simulink model "pulse_heating_official_spine_v04_git_recovery"  (R2025b)
settings: Solver=VariableStepAuto  StartTime=0.0  StopTime=0.001  RelTol=1e-3
PreLoadFcn:
  | addpath('C:\Users\ADMIN\Documents\MATLAB\Examples\R2025b\simscapeelectrical\BatteryThermalManagementExample');
  | addpath('C:\Users\ADMIN\Documents\MATLAB\Examples\R2025b\mcb\SIUnitsExample');
  | addpath('C:\Users\ADMIN\Documents\MATLAB\Examples\R2025b\simscapeelectrical\PMSMDriveThermalExample');
  | load_system('PMSMDriveThermal');
  | set_param('PMSMDriveThermal','SimscapeLogType','none','SimscapeLogSimulationStatistics','off');
  | set_param('PMSMDriveThermal','Dirty','off');
InitFcn:
  | addpath('C:\Users\ADMIN\Documents\MATLAB\Examples\R2025b\simscapeelectrical\BatteryThermalManagementExample');
  | addpath('C:\Users\ADMIN\Documents\MATLAB\Examples\R2025b\mcb\SIUnitsExample');
  | addpath('C:\Users\ADMIN\Documents\MATLAB\Examples\R2025b\simscapeelectrical\PMSMDriveThermalExample');
  | load_system('PMSMDriveThermal');
  | PMSMDriveThermalData;
  | mcb_pmsm_foc_qep_f28379d_SIUnit_data;
  | bw_i = (PI_params.Kp_i + pmsm.Rs) / pmsm.Ld;
  | pmsm.Rs = Rs; pmsm.Ld = Ld; pmsm.Lq = Lq; pmsm.p = N; pmsm.FluxPM = PM;
  | pmsm.J = J; pmsm.Ke = PM*N; pmsm.Kt = 1.5*N*PM;
  | PI_params.Kp_i = bw_i * Ld - Rs; PI_params.Ki_i = bw_i * Rs; PI_params.Ti_i = 1/bw_i;
  | PI_params.Kp_id = PI_params.Kp_i; PI_params.Ki_id = PI_params.Ki_i; PI_params.Ti_id = PI_params.Ti_i;
  | inverter.V_dc = 70; dataType = 'double';
  | BatteryThermalManagementInitialization;
  | ambient=263.15; coolantTemp=263.15; cellT_ini=ambient*ones(1,Ns*Np); cellT_ini4=ambient*ones(1,Ns4*Np4);
model workspace (MAT data in the model file):
  control_status_v4d2_partial_duty_code = 6
  diagnostic_frequency_Hz = 50
  drive_status_v4d2_partial_current_code = 6
  kpi_status_v4d2_partial_numeric_code = 6
  kpi_value_unknown = nan
  limit_factor_unknown_code = 99
  limit_margin_unknown_value = nan
  limit_status_v4c_code = 5
  pulse_command_status_code = 6
  pulse_duty_percent = 50
  pulse_id_amplitude_A = 1
  pulse_iq_amplitude_A = 0
  pulse_mode_code = 4
  pulse_phase_delay_s = 0
undefined symbols (not defined in the file): DiscIntNeverNeededParam, f_losses, Flowrate_vec, fsw, Isc_losses, losses_oc, losses_sc, N, PM, Rs, Ts, Tsc
libraries: fl_lib x36, nesl_utility x33, ee_lib x9, mcbcontrolslib x5, mcbeeMathTransformLib x3, slpidlib x2, simulink x1
(part 2 of 4)

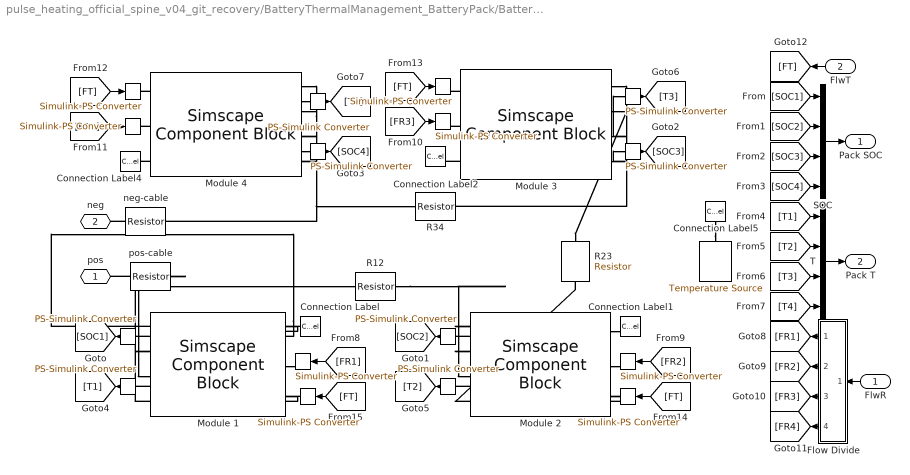
== system pulse_heating_official_spine_v04_git_recovery/BatteryThermalManagement_BatteryPack/Battery_pack ==
  FlwR : Inport
  FlwT : Inport  Port=2
  " " : nesl_utility/PS-Simulink Converter  PhysicalDomain=network_engine_domain  SubClassName=ps_output  LeftPortType=input  RightPortType=output  PseudoPeriodic=off  Frequencies=[]  VectorFormat=1-D array  Unit=inherit  AffineConversion=off
  "  " : nesl_utility/PS-Simulink Converter  PhysicalDomain=network_engine_domain  SubClassName=ps_output  LeftPortType=input  RightPortType=output  PseudoPeriodic=off  Frequencies=[]  VectorFormat=1-D array  Unit=inherit  AffineConversion=off
  "   " : nesl_utility/PS-Simulink Converter  PhysicalDomain=network_engine_domain  SubClassName=ps_output  LeftPortType=input  RightPortType=output  PseudoPeriodic=off  Frequencies=[]  VectorFormat=1-D array  Unit=inherit  AffineConversion=off
  "    " : nesl_utility/Simulink-PS Converter  PhysicalDomain=network_engine_domain  SubClassName=ps_input  LeftPortType=input  RightPortType=output  PseudoPeriodic=off  Frequencies=[]  NoiseDistribution=none  NoiseParameters=[]  Unit=1  AffineConversion=off  FilteringAndDerivatives=filter  SimscapeFilterOrder=1  InputFilterTimeConstant=0.01  UdotUserProvided=0
  "     " : fl_lib/Thermal/Thermal Sources/Temperature Source  temperature=ambient K
  "      " : nesl_utility/PS-Simulink Converter  PhysicalDomain=network_engine_domain  SubClassName=ps_output  LeftPortType=input  RightPortType=output  PseudoPeriodic=off  Frequencies=[]  VectorFormat=1-D array  Unit=inherit  AffineConversion=off
  "       " : nesl_utility/Simulink-PS Converter  PhysicalDomain=network_engine_domain  SubClassName=ps_input  LeftPortType=input  RightPortType=output  PseudoPeriodic=off  Frequencies=[]  NoiseDistribution=none  NoiseParameters=[]  Unit=1  AffineConversion=off  FilteringAndDerivatives=filter  SimscapeFilterOrder=1  InputFilterTimeConstant=0.01  UdotUserProvided=0
  "         " : nesl_utility/PS-Simulink Converter  PhysicalDomain=network_engine_domain  SubClassName=ps_output  LeftPortType=input  RightPortType=output  PseudoPeriodic=off  Frequencies=[]  VectorFormat=1-D array  Unit=inherit  AffineConversion=off
  "          " : nesl_utility/PS-Simulink Converter  PhysicalDomain=network_engine_domain  SubClassName=ps_output  LeftPortType=input  RightPortType=output  PseudoPeriodic=off  Frequencies=[]  VectorFormat=1-D array  Unit=inherit  AffineConversion=off
  "           " : nesl_utility/Simulink-PS Converter  PhysicalDomain=network_engine_domain  SubClassName=ps_input  LeftPortType=input  RightPortType=output  PseudoPeriodic=off  Frequencies=[]  NoiseDistribution=none  NoiseParameters=[]  Unit=1  AffineConversion=off  FilteringAndDerivatives=filter  SimscapeFilterOrder=1  InputFilterTimeConstant=0.01  UdotUserProvided=0
  "            " : nesl_utility/PS-Simulink Converter  PhysicalDomain=network_engine_domain  SubClassName=ps_output  LeftPortType=input  RightPortType=output  PseudoPeriodic=off  Frequencies=[]  VectorFormat=1-D array  Unit=inherit  AffineConversion=off
  "              " : nesl_utility/Simulink-PS Converter  PhysicalDomain=network_engine_domain  SubClassName=ps_input  LeftPortType=input  RightPortType=output  PseudoPeriodic=off  Frequencies=[]  NoiseDistribution=none  NoiseParameters=[]  Unit=1  AffineConversion=off  FilteringAndDerivatives=filter  SimscapeFilterOrder=1  InputFilterTimeConstant=0.01  UdotUserProvided=0
  "               " : nesl_utility/Simulink-PS Converter  PhysicalDomain=network_engine_domain  SubClassName=ps_input  LeftPortType=input  RightPortType=output  PseudoPeriodic=off  Frequencies=[]  NoiseDistribution=none  NoiseParameters=[]  Unit=1  AffineConversion=off  FilteringAndDerivatives=filter  SimscapeFilterOrder=1  InputFilterTimeConstant=0.01  UdotUserProvided=0
  "                      " : nesl_utility/Simulink-PS Converter  PhysicalDomain=network_engine_domain  SubClassName=ps_input  LeftPortType=input  RightPortType=output  PseudoPeriodic=off  Frequencies=[]  NoiseDistribution=none  NoiseParameters=[]  Unit=1  AffineConversion=off  FilteringAndDerivatives=filter  SimscapeFilterOrder=1  InputFilterTimeConstant=0.01  UdotUserProvided=0
  "                                      " : nesl_utility/PS-Simulink Converter  PhysicalDomain=network_engine_domain  SubClassName=ps_output  LeftPortType=input  RightPortType=output  PseudoPeriodic=off  Frequencies=[]  VectorFormat=1-D array  Unit=inherit  AffineConversion=off
  "                                           " : nesl_utility/Simulink-PS Converter  PhysicalDomain=network_engine_domain  SubClassName=ps_input  LeftPortType=input  RightPortType=output  PseudoPeriodic=off  Frequencies=[]  NoiseDistribution=none  NoiseParameters=[]  Unit=1  AffineConversion=off  FilteringAndDerivatives=filter  SimscapeFilterOrder=1  InputFilterTimeConstant=0.01  UdotUserProvided=0
  "                                                  " : nesl_utility/Simulink-PS Converter  PhysicalDomain=network_engine_domain  SubClassName=ps_input  LeftPortType=input  RightPortType=output  PseudoPeriodic=off  Frequencies=[]  NoiseDistribution=none  NoiseParameters=[]  Unit=1  AffineConversion=off  FilteringAndDerivatives=filter  SimscapeFilterOrder=1  InputFilterTimeConstant=0.01  UdotUserProvided=0
  "                        Flow Divide" : Subsystem
  Connection Label{,1..2,4..5} (5 alike) : ConnectionLabel  Label=Amb
  Module 1 : SimscapeComponentBlock  SourceFile=BatteryModule  ComponentPath=BatteryModule  ComponentVariants="[\"BatteryModule\"]"  ComponentVariantNames="[\"BatteryModule\"]"  ClassName=BatteryModule  SchemaVersion=1  LUTpointsTemp=T_vec K  cellAH=AH A*hr  LUTpointsSOC=SOC_vec  LUTpointsFlowrate=Flowrate_vec kg/s  V0_mat=V0_mat V  prm_dir=simscape.enum.tablebattery.prm_dir.noCurrentDirectionality  R0_mat=R0_mat Ohm  R0_dis_mat=[.03, .015, .002; .04, .017, .008; .039, .012, .006; .027, .013, .021] Ohm  R0_ch_mat=[.03, .015, .002; .04, .017, .008; .039, .012, .006; .027, .013, .021] Ohm  prm_leak=simscape.enum.tablebattery.prm_leak.disabled  Rleak_vec=Rleak Ohm  extrapolation_option=simscape.enum.extrapolation.nearest  prm_dyn=simscape.enum.tablebattery.prm_dyn.rc2  R1_mat=R1_mat Ohm  tau1_mat=Tau1_mat s  R2_mat=R2_mat Ohm  tau2_mat=Tau2_mat s  R3_mat=[.014, .382, .407; .028, .006, .007; .014, .007, .006; .333, .956, .912] Ohm  tau3_mat=[1, 44, 5644; 11, 24, 506; 2, 14, 330; 3310, 13419, 30216] s  R4_mat=[.014, .382, .407; .028, .006, .007; .014, .007, .006; .333, .956, .912] Ohm  tau4_mat=[1, 44, 5644; 11, 24, 506; 2, 14, 330; 3310, 13419, 30216] s  R5_mat=[.014, .382, .407; .028, .006, .007; .014, .007, .006; .333, .956, .912] Ohm  tau5_mat=[1, 44, 5644; 11, 24, 506; 2, 14, 330; 3310, 13419, 30216] s  prm_fade=simscape.enum.tablebattery.prm_fade.equations  N0=Ndisc  dV0=delV0  dR0=delR0  dAH=delAH  dRleak=delLeak  dR1=delR1  dR2=delR2  dR3=0  dR4=0  dR5=0  N0vec=[100, 200, 300]  Tfadevec=[298.15, 323.15] K  dV0vec=[0, 0, 0]  dR0vec=[0, 0, 0]  dAHvec=[0, 0, 0]  dRleakvec=[0, 0, 0]  dR1vec=[0, 0, 0]  dR2vec=[0, 0, 0]  dR3vec=[0, 0, 0]  dR4vec=[0, 0, 0]  dR5vec=[0, 0, 0]  dV0mat=[0, 0; 0, 0; 0, 0]  dR0mat=[0, 0; 0, 0; 0, 0]  dAHmat=[0, 0; 0, 0; 0, 0]  dRleakmat=[0, 0; 0, 0; 0, 0]  dR1mat=[0, 0; 0, 0; 0, 0]  dR2mat=[0, 0; 0, 0; 0, 0]  dR3mat=[0, 0; 0, 0; 0, 0]  dR4mat=[0, 0; 0, 0; 0, 0]  dR5mat=[0, 0; 0, 0; 0, 0]  cellThermalMass=MdotCp J/K  cellThermalCond=K_cell W/(m*K)  cellHeatTrCoeff=h_cell W/(m^2*K)  Ns=Ns  Np=Np  cellTypeSelection=BatteryTypeSelection.Pouch  cellHeight=cell_H m  cellWidth=cell_W m  cellThickness=cell_T m  cellDiameter=0.018 m  cellCylinLine=3  moduleExternalR=Rext Ohm  moduleCellBalancing=BatteryCellBalancingEnum.None  passiveShuntR=shuntR Ohm  passiveSWclosedR=swClosedR Ohm  passiveSWopenCond=swOpenC 1/Ohm  passiveSWthreshold=swThreshold  moduleCooling=coolantQ W/K  moduleExtHeat=extHeat W  cellTemp=cellT_ini K  cellSOC=cellSOC_ini  moduleCellAHpercentVar=AhrVar  moduleCellLeakPercentVar=RleakVar
      settings: CopyFcn=simscape.sscblock.internal.componentBlockCallback(gcbh,'COPY')  PreCopyFcn=simscape.sscblock.internal.componentBlockCallback(gcbh,'PRECOPY')  PreDeleteFcn=simscape.sscblock.internal.componentBlockCallback(gcbh,'PREDELETE')  InternalSimscapePortConfiguration="{\"Bottom\":[],\"Left\":[{\"id\":\"outputCellSOC\",\"label\":\"SOC\",\"type\":\"output\"},{\"id\":\"outputCellTemp\",\"label\":\"Temp\",\"type\":\"output\"}],\"Right\":[{\"id\":\"H\",\"label\":\"Amb\",\"type\":\"foundation.thermal.thermal\"},{\"id\":\"frac\",\"label\":\"FlwR\",\"type\":\"input\"},{\"id\":\"delT\",\"label\":\"FlwT\",\"type\":\"input\"}],\"Top\":[{\"id\":\"p\",\"label\":\"pos\",\"type\":\"foundation.electrical.electrical\"},{\"id\":\"n\",\"label\":\"neg\",\"type\":\"foundation.electrical.electrical\"}]}"
      mask Type: Battery Module
  Module 2 : SimscapeComponentBlock  SourceFile=BatteryModule  ComponentPath=BatteryModule  ComponentVariants="[\"BatteryModule\"]"  ComponentVariantNames="[\"BatteryModule\"]"  ClassName=BatteryModule  SchemaVersion=1  LUTpointsTemp=T_vec K  cellAH=AH A*hr  LUTpointsSOC=SOC_vec  LUTpointsFlowrate=Flowrate_vec kg/s  V0_mat=V0_mat V  prm_dir=simscape.enum.tablebattery.prm_dir.noCurrentDirectionality  R0_mat=R0_mat Ohm  R0_dis_mat=[.03, .015, .002; .04, .017, .008; .039, .012, .006; .027, .013, .021] Ohm  R0_ch_mat=[.03, .015, .002; .04, .017, .008; .039, .012, .006; .027, .013, .021] Ohm  prm_leak=simscape.enum.tablebattery.prm_leak.disabled  Rleak_vec=Rleak Ohm  extrapolation_option=simscape.enum.extrapolation.nearest  prm_dyn=simscape.enum.tablebattery.prm_dyn.rc2  R1_mat=R1_mat Ohm  tau1_mat=Tau1_mat s  R2_mat=R2_mat Ohm  tau2_mat=Tau2_mat s  R3_mat=[.014, .382, .407; .028, .006, .007; .014, .007, .006; .333, .956, .912] Ohm  tau3_mat=[1, 44, 5644; 11, 24, 506; 2, 14, 330; 3310, 13419, 30216] s  R4_mat=[.014, .382, .407; .028, .006, .007; .014, .007, .006; .333, .956, .912] Ohm  tau4_mat=[1, 44, 5644; 11, 24, 506; 2, 14, 330; 3310, 13419, 30216] s  R5_mat=[.014, .382, .407; .028, .006, .007; .014, .007, .006; .333, .956, .912] Ohm  tau5_mat=[1, 44, 5644; 11, 24, 506; 2, 14, 330; 3310, 13419, 30216] s  prm_fade=simscape.enum.tablebattery.prm_fade.equations  N0=Ndisc  dV0=delV0  dR0=delR0  dAH=delAH  dRleak=delLeak  dR1=delR1  dR2=delR2  dR3=0  dR4=0  dR5=0  N0vec=[100, 200, 300]  Tfadevec=[298.15, 323.15] K  dV0vec=[0, 0, 0]  dR0vec=[0, 0, 0]  dAHvec=[0, 0, 0]  dRleakvec=[0, 0, 0]  dR1vec=[0, 0, 0]  dR2vec=[0, 0, 0]  dR3vec=[0, 0, 0]  dR4vec=[0, 0, 0]  dR5vec=[0, 0, 0]  dV0mat=[0, 0; 0, 0; 0, 0]  dR0mat=[0, 0; 0, 0; 0, 0]  dAHmat=[0, 0; 0, 0; 0, 0]  dRleakmat=[0, 0; 0, 0; 0, 0]  dR1mat=[0, 0; 0, 0; 0, 0]  dR2mat=[0, 0; 0, 0; 0, 0]  dR3mat=[0, 0; 0, 0; 0, 0]  dR4mat=[0, 0; 0, 0; 0, 0]  dR5mat=[0, 0; 0, 0; 0, 0]  cellThermalMass=MdotCp J/K  cellThermalCond=K_cell W/(m*K)  cellHeatTrCoeff=h_cell W/(m^2*K)  Ns=Ns  Np=Np  cellTypeSelection=BatteryTypeSelection.Pouch  cellHeight=cell_H m  cellWidth=cell_W m  cellThickness=cell_T m  cellDiameter=0.018 m  cellCylinLine=3  moduleExternalR=Rext Ohm  moduleCellBalancing=BatteryCellBalancingEnum.None  passiveShuntR=shuntR Ohm  passiveSWclosedR=swClosedR Ohm  passiveSWopenCond=swOpenC 1/Ohm  passiveSWthreshold=swThreshold  moduleCooling=coolantQ W/K  moduleExtHeat=extHeat W  cellTemp=cellT_ini K  cellSOC=cellSOC_ini  moduleCellAHpercentVar=AhrVar  moduleCellLeakPercentVar=RleakVar
      settings: CopyFcn=simscape.sscblock.internal.componentBlockCallback(gcbh,'COPY')  PreCopyFcn=simscape.sscblock.internal.componentBlockCallback(gcbh,'PRECOPY')  PreDeleteFcn=simscape.sscblock.internal.componentBlockCallback(gcbh,'PREDELETE')  InternalSimscapePortConfiguration="{\"Bottom\":[],\"Left\":[{\"id\":\"outputCellSOC\",\"label\":\"SOC\",\"type\":\"output\"},{\"id\":\"outputCellTemp\",\"label\":\"Temp\",\"type\":\"output\"}],\"Right\":[{\"id\":\"H\",\"label\":\"Amb\",\"type\":\"foundation.thermal.thermal\"},{\"id\":\"frac\",\"label\":\"FlwR\",\"type\":\"input\"},{\"id\":\"delT\",\"label\":\"FlwT\",\"type\":\"input\"}],\"Top\":[{\"id\":\"p\",\"label\":\"pos\",\"type\":\"foundation.electrical.electrical\"},{\"id\":\"n\",\"label\":\"neg\",\"type\":\"foundation.electrical.electrical\"}]}"
      mask Type: Battery Module
  Module 3 : SimscapeComponentBlock  SourceFile=BatteryModule  ComponentPath=BatteryModule  ComponentVariants="[\"BatteryModule\"]"  ComponentVariantNames="[\"BatteryModule\"]"  ClassName=BatteryModule  SchemaVersion=1  LUTpointsTemp=T_vec K  cellAH=AH A*hr  LUTpointsSOC=SOC_vec  LUTpointsFlowrate=Flowrate_vec kg/s  V0_mat=V0_mat V  prm_dir=simscape.enum.tablebattery.prm_dir.noCurrentDirectionality  R0_mat=R0_mat Ohm  R0_dis_mat=[.03, .015, .002; .04, .017, .008; .039, .012, .006; .027, .013, .021] Ohm  R0_ch_mat=[.03, .015, .002; .04, .017, .008; .039, .012, .006; .027, .013, .021] Ohm  prm_leak=simscape.enum.tablebattery.prm_leak.disabled  Rleak_vec=Rleak Ohm  extrapolation_option=simscape.enum.extrapolation.nearest  prm_dyn=simscape.enum.tablebattery.prm_dyn.rc2  R1_mat=R1_mat Ohm  tau1_mat=Tau1_mat s  R2_mat=R2_mat Ohm  tau2_mat=Tau2_mat s  R3_mat=[.014, .382, .407; .028, .006, .007; .014, .007, .006; .333, .956, .912] Ohm  tau3_mat=[1, 44, 5644; 11, 24, 506; 2, 14, 330; 3310, 13419, 30216] s  R4_mat=[.014, .382, .407; .028, .006, .007; .014, .007, .006; .333, .956, .912] Ohm  tau4_mat=[1, 44, 5644; 11, 24, 506; 2, 14, 330; 3310, 13419, 30216] s  R5_mat=[.014, .382, .407; .028, .006, .007; .014, .007, .006; .333, .956, .912] Ohm  tau5_mat=[1, 44, 5644; 11, 24, 506; 2, 14, 330; 3310, 13419, 30216] s  prm_fade=simscape.enum.tablebattery.prm_fade.equations  N0=Ndisc  dV0=delV0  dR0=delR0  dAH=delAH  dRleak=delLeak  dR1=delR1  dR2=delR2  dR3=0  dR4=0  dR5=0  N0vec=[100, 200, 300]  Tfadevec=[298.15, 323.15] K  dV0vec=[0, 0, 0]  dR0vec=[0, 0, 0]  dAHvec=[0, 0, 0]  dRleakvec=[0, 0, 0]  dR1vec=[0, 0, 0]  dR2vec=[0, 0, 0]  dR3vec=[0, 0, 0]  dR4vec=[0, 0, 0]  dR5vec=[0, 0, 0]  dV0mat=[0, 0; 0, 0; 0, 0]  dR0mat=[0, 0; 0, 0; 0, 0]  dAHmat=[0, 0; 0, 0; 0, 0]  dRleakmat=[0, 0; 0, 0; 0, 0]  dR1mat=[0, 0; 0, 0; 0, 0]  dR2mat=[0, 0; 0, 0; 0, 0]  dR3mat=[0, 0; 0, 0; 0, 0]  dR4mat=[0, 0; 0, 0; 0, 0]  dR5mat=[0, 0; 0, 0; 0, 0]  cellThermalMass=MdotCp J/K  cellThermalCond=K_cell W/(m*K)  cellHeatTrCoeff=h_cell W/(m^2*K)  Ns=Ns  Np=Np  cellTypeSelection=BatteryTypeSelection.Pouch  cellHeight=cell_H m  cellWidth=cell_W m  cellThickness=cell_T m  cellDiameter=0.018 m  cellCylinLine=3  moduleExternalR=Rext Ohm  moduleCellBalancing=BatteryCellBalancingEnum.None  passiveShuntR=shuntR Ohm  passiveSWclosedR=swClosedR Ohm  passiveSWopenCond=swOpenC 1/Ohm  passiveSWthreshold=swThreshold  moduleCooling=coolantQ W/K  moduleExtHeat=extHeat W  cellTemp=cellT_ini K  cellSOC=cellSOC_ini  moduleCellAHpercentVar=AhrVar  moduleCellLeakPercentVar=RleakVar
      settings: CopyFcn=simscape.sscblock.internal.componentBlockCallback(gcbh,'COPY')  PreCopyFcn=simscape.sscblock.internal.componentBlockCallback(gcbh,'PRECOPY')  PreDeleteFcn=simscape.sscblock.internal.componentBlockCallback(gcbh,'PREDELETE')  InternalSimscapePortConfiguration="{\"Bottom\":[],\"Left\":[{\"id\":\"outputCellSOC\",\"label\":\"SOC\",\"type\":\"output\"},{\"id\":\"outputCellTemp\",\"label\":\"Temp\",\"type\":\"output\"}],\"Right\":[{\"id\":\"H\",\"label\":\"Amb\",\"type\":\"foundation.thermal.thermal\"},{\"id\":\"frac\",\"label\":\"FlwR\",\"type\":\"input\"},{\"id\":\"delT\",\"label\":\"FlwT\",\"type\":\"input\"}],\"Top\":[{\"id\":\"p\",\"label\":\"pos\",\"type\":\"foundation.electrical.electrical\"},{\"id\":\"n\",\"label\":\"neg\",\"type\":\"foundation.electrical.electrical\"}]}"
      mask Type: Battery Module
  Module 4 : SimscapeComponentBlock  SourceFile=BatteryModule  ComponentPath=BatteryModule  ComponentVariants="[\"BatteryModule\"]"  ComponentVariantNames="[\"BatteryModule\"]"  ClassName=BatteryModule  SchemaVersion=1  LUTpointsTemp=T_vec K  cellAH=AH A*hr  LUTpointsSOC=SOC_vec  LUTpointsFlowrate=Flowrate_vec kg/s  V0_mat=V0_mat V  prm_dir=simscape.enum.tablebattery.prm_dir.noCurrentDirectionality  R0_mat=R0_mat Ohm  R0_dis_mat=[.03, .015, .002; .04, .017, .008; .039, .012, .006; .027, .013, .021] Ohm  R0_ch_mat=[.03, .015, .002; .04, .017, .008; .039, .012, .006; .027, .013, .021] Ohm  prm_leak=simscape.enum.tablebattery.prm_leak.disabled  Rleak_vec=Rleak Ohm  extrapolation_option=simscape.enum.extrapolation.nearest  prm_dyn=simscape.enum.tablebattery.prm_dyn.rc2  R1_mat=R1_mat Ohm  tau1_mat=Tau1_mat s  R2_mat=R2_mat Ohm  tau2_mat=Tau2_mat s  R3_mat=[.014, .382, .407; .028, .006, .007; .014, .007, .006; .333, .956, .912] Ohm  tau3_mat=[1, 44, 5644; 11, 24, 506; 2, 14, 330; 3310, 13419, 30216] s  R4_mat=[.014, .382, .407; .028, .006, .007; .014, .007, .006; .333, .956, .912] Ohm  tau4_mat=[1, 44, 5644; 11, 24, 506; 2, 14, 330; 3310, 13419, 30216] s  R5_mat=[.014, .382, .407; .028, .006, .007; .014, .007, .006; .333, .956, .912] Ohm  tau5_mat=[1, 44, 5644; 11, 24, 506; 2, 14, 330; 3310, 13419, 30216] s  prm_fade=simscape.enum.tablebattery.prm_fade.equations  N0=Ndisc  dV0=delV0  dR0=delR0  dAH=delAH  dRleak=delLeak  dR1=delR1  dR2=delR2  dR3=0  dR4=0  dR5=0  N0vec=[100, 200, 300]  Tfadevec=[298.15, 323.15] K  dV0vec=[0, 0, 0]  dR0vec=[0, 0, 0]  dAHvec=[0, 0, 0]  dRleakvec=[0, 0, 0]  dR1vec=[0, 0, 0]  dR2vec=[0, 0, 0]  dR3vec=[0, 0, 0]  dR4vec=[0, 0, 0]  dR5vec=[0, 0, 0]  dV0mat=[0, 0; 0, 0; 0, 0]  dR0mat=[0, 0; 0, 0; 0, 0]  dAHmat=[0, 0; 0, 0; 0, 0]  dRleakmat=[0, 0; 0, 0; 0, 0]  dR1mat=[0, 0; 0, 0; 0, 0]  dR2mat=[0, 0; 0, 0; 0, 0]  dR3mat=[0, 0; 0, 0; 0, 0]  dR4mat=[0, 0; 0, 0; 0, 0]  dR5mat=[0, 0; 0, 0; 0, 0]  cellThermalMass=MdotCp J/K  cellThermalCond=K_cell W/(m*K)  cellHeatTrCoeff=h_cell W/(m^2*K)  Ns=Ns4  Np=Np4  cellTypeSelection=BatteryTypeSelection.Pouch  cellHeight=cell_H m  cellWidth=cell_W m  cellThickness=cell_T m  cellDiameter=0.018 m  cellCylinLine=3  moduleExternalR=Rext4 Ohm  moduleCellBalancing=BatteryCellBalancingEnum.None  passiveShuntR=shuntR Ohm  passiveSWclosedR=swClosedR Ohm  passiveSWopenCond=swOpenC 1/Ohm  passiveSWthreshold=swThreshold  moduleCooling=coolantQ4 W/K  moduleExtHeat=extHeat4 W  cellTemp=cellT_ini4 K  cellSOC=cellSOC_ini4  moduleCellAHpercentVar=AhrVar4  moduleCellLeakPercentVar=RleakVar
      settings: CopyFcn=simscape.sscblock.internal.componentBlockCallback(gcbh,'COPY')  PreCopyFcn=simscape.sscblock.internal.componentBlockCallback(gcbh,'PRECOPY')  PreDeleteFcn=simscape.sscblock.internal.componentBlockCallback(gcbh,'PREDELETE')  InternalSimscapePortConfiguration="{\"Bottom\":[],\"Left\":[{\"id\":\"outputCellSOC\",\"label\":\"SOC\",\"type\":\"output\"},{\"id\":\"outputCellTemp\",\"label\":\"Temp\",\"type\":\"output\"}],\"Right\":[{\"id\":\"H\",\"label\":\"Amb\",\"type\":\"foundation.thermal.thermal\"},{\"id\":\"frac\",\"label\":\"FlwR\",\"type\":\"input\"},{\"id\":\"delT\",\"label\":\"FlwT\",\"type\":\"input\"}],\"Top\":[{\"id\":\"p\",\"label\":\"pos\",\"type\":\"foundation.electrical.electrical\"},{\"id\":\"n\",\"label\":\"neg\",\"type\":\"foundation.electrical.electrical\"}]}"
      mask Type: Battery Module
  R12 : fl_lib/Electrical/Electrical Elements/Resistor  R=0.001 Ohm  i_specify=off  i_priority=None  i=0 A  i_nominal_specify=off  i_nominal_value=1  i_nominal_unit=A  v_specify=off  v_priority=None  v=0 V  v_nominal_specify=off  v_nominal_value=1  v_nominal_unit=V
  R23 : fl_lib/Electrical/Electrical Elements/Resistor  R=0.001 Ohm  i_specify=off  i_priority=None  i=0 A  i_nominal_specify=off  i_nominal_value=1  i_nominal_unit=A  v_specify=off  v_priority=None  v=0 V  v_nominal_specify=off  v_nominal_value=1  v_nominal_unit=V
  R34 : fl_lib/Electrical/Electrical Elements/Resistor  R=0.001 Ohm  i_specify=off  i_priority=None  i=0 A  i_nominal_specify=off  i_nominal_value=1  i_nominal_unit=A  v_specify=off  v_priority=None  v=0 V  v_nominal_specify=off  v_nominal_value=1  v_nominal_unit=V
  SOC : Concatenate  NumInputs=4
  T : Concatenate  NumInputs=4
  neg-cable : fl_lib/Electrical/Electrical Elements/Resistor  R=0.001 Ohm  i_specify=off  i_priority=None  i=0 A  i_nominal_specify=off  i_nominal_value=1  i_nominal_unit=A  v_specify=off  v_priority=None  v=0 V  v_nominal_specify=off  v_nominal_value=1  v_nominal_unit=V
  pos-cable : fl_lib/Electrical/Electrical Elements/Resistor  R=0.001 Ohm  i_specify=off  i_priority=None  i=0 A  i_nominal_specify=off  i_nominal_value=1  i_nominal_unit=A  v_specify=off  v_priority=None  v=0 V  v_nominal_specify=off  v_nominal_value=1  v_nominal_unit=V
  pos : PMIOPort  Side=Left
  neg : PMIOPort  Port=2  Side=Right
  Pack SOC : Outport
  Pack T : Outport  Port=2
  wires:
  "                        Flow Divide"/4(Out4) -> [FR4]
  "                        Flow Divide"/3(Out3) -> [FR3]
  "                        Flow Divide"/2(Out2) -> [FR2]
  "                        Flow Divide"/1(Out1) -> [FR1]
  FlwR/1 -> "                        Flow Divide"/1(In1)
  T/1 -> Pack T/1
  SOC/1 -> Pack SOC/1
  FlwT/1 -> [FT]
  [FT] -> "                                           "/1
  [FT] -> "                                                  "/1
  [FT] -> "              "/1
  [FT] -> "               "/1
  [FR4] -> "           "/1
  [FR3] -> "                      "/1
  [FR2] -> "       "/1
  [FR1] -> "    "/1
  "                                      "/1 -> [T4]
  "         "/1 -> [T3]
  "   "/1 -> [T2]
  " "/1 -> [T1]
  [T1] -> T/1
  [T2] -> T/2
  [T4] -> T/4
  [T3] -> T/3
  [SOC4] -> SOC/4
  [SOC3] -> SOC/3
  [SOC2] -> SOC/2
  [SOC1] -> SOC/1
  "            "/1 -> [SOC4]
  "          "/1 -> [SOC3]
  "      "/1 -> [SOC2]
  "  "/1 -> [SOC1]
  connections:
  pos-cable/RConn1 -- Module 1/LConn3
  pos-cable/LConn1 -- pos/RConn1
  Module 4/LConn4 -- neg-cable/LConn1
  neg-cable/RConn1 -- neg/RConn1
  Module 2/LConn4 -- R23/LConn1
  Module 3/LConn3 -- R23/RConn1
  Module 4/LConn3 -- R34/RConn1
  Module 3/LConn4 -- R34/LConn1
  R12/RConn1 -- Module 2/LConn3
  Module 1/LConn4 -- R12/LConn1
  "                                           "/RConn1 -- Module 1/RConn3
  "                                                  "/RConn1 -- Module 2/RConn3
  Module 1/RConn2 -- "    "/RConn1
  Connection Label5/LConn1 -- "     "/LConn1
  Module 4/RConn1 -- Connection Label4/LConn1
  Module 3/RConn1 -- Connection Label2/LConn1
  Module 2/RConn1 -- Connection Label1/LConn1
  Connection Label/LConn1 -- Module 1/RConn1
  Module 3/LConn2 -- "         "/LConn1
  Module 3/LConn1 -- "          "/LConn1
  Module 1/LConn1 -- "  "/LConn1
  Module 2/RConn2 -- "       "/RConn1
  Module 3/RConn2 -- "                      "/RConn1
  Module 4/RConn3 -- "               "/RConn1
  Module 2/LConn2 -- "   "/LConn1
  Module 4/LConn2 -- "                                      "/LConn1
  Module 2/LConn1 -- "      "/LConn1
  Module 4/LConn1 -- "            "/LConn1
  Module 1/LConn2 -- " "/LConn1
  Module 4/RConn2 -- "           "/RConn1
  Module 3/RConn3 -- "              "/RConn1

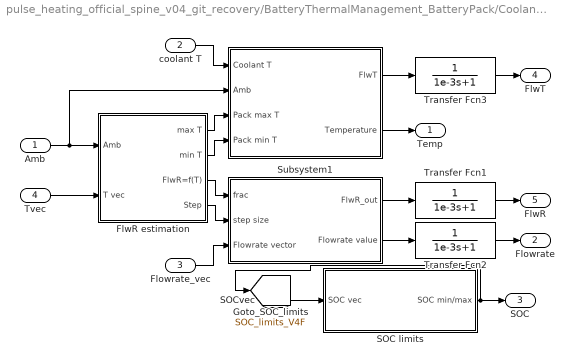
== system pulse_heating_official_spine_v04_git_recovery/BatteryThermalManagement_BatteryPack/Coolant_control ==
  Amb : Inport
  coolant T : Inport  Port=2
  Flowrate_vec : Inport  Port=3
  Tvec : Inport  Port=4
  SOCvec : Inport  Port=5
  "   " : Subsystem
  FlwR estimation : Subsystem
  SOC limits : Subsystem
  Subsystem1 : Subsystem
  Transfer Fcn1 : TransferFcn  Denominator=[1e-3 1]
  Transfer Fcn2 : TransferFcn  Denominator=[1e-3 1]
  Transfer Fcn3 : TransferFcn  Denominator=[1e-3 1]
  Temp : Outport
  Flowrate : Outport  Port=2
  SOC : Outport  Port=3
  FlwT : Outport  Port=4
  FlwR : Outport  Port=5
  tag scope: SOC_limits_V4F=global
  wires:
  Amb/1 -> "   "/2(Amb), FlwR estimation/1(Amb)
  Flowrate_vec/1 -> Subsystem1/3(Flowrate vector)
  Subsystem1/2(Flowrate value) -> Transfer Fcn2/1
  Subsystem1/1(FlwR_out) -> Transfer Fcn1/1
  FlwR estimation/4(Step) -> Subsystem1/2(step size)
  FlwR estimation/3(FlwR=f(T)) -> Subsystem1/1(frac)
  "   "/2(Temperature) -> Temp/1
  "   "/1(FlwT) -> Transfer Fcn3/1
  FlwR estimation/2(min T) -> "   "/4(Pack min T)
  FlwR estimation/1(max T) -> "   "/3(Pack max T)
  coolant T/1 -> "   "/1(Coolant T)
  Tvec/1 -> FlwR estimation/2(T vec)
  SOC limits/1(SOC min/max) -> SOC/1, [SOC_limits_V4F]
  SOCvec/1 -> SOC limits/1(SOC vec)
  Transfer Fcn3/1 -> FlwT/1
  Transfer Fcn2/1 -> Flowrate/1
  Transfer Fcn1/1 -> FlwR/1

== system pulse_heating_official_spine_v04_git_recovery/MCB_SIUnits_FOC_Controller/Control_System ==
  Iab_meas : Inport
  Pos : Inport  Port=2
  EnClosedLoop : Inport  Port=3
  Idq_ref : Inport  Port=4
  Closed Loop Control : Subsystem
  NOT : Logic  Operator=NOT  IconShape=distinctive  AllPortsSameDT=off  OutDataTypeStr=boolean
  Open Loop Start-Up : Subsystem
  Switch4 : Switch  Threshold=0.5  OutDataTypeStr=Inherit: Inherit via back propagation  RndMeth=Simplest  SaturateOnIntegerOverflow=off  InputSameDT=off
  Duty_abc : Outport  VectorParamsAs1DForOutWhenUnconnected=off
  Idq_debug : Outport  Port=2  VectorParamsAs1DForOutWhenUnconnected=off
  wires:
  Closed Loop Control/1(Idq_debug) -> Idq_debug/1
  Switch4/1 -> Duty_abc/1  "PWM_Duty_Cycles"
  NOT/1 -> Open Loop Start-Up/Enable
  Closed Loop Control/2(Duty_abc) -> Switch4/1
  Idq_ref/1 -> Closed Loop Control/3(Idq_ref)
  Pos/1 -> Closed Loop Control/2(Pos)
  Iab_meas/1 -> Closed Loop Control/1(Iab_meas)
  Open Loop Start-Up/1(Duty_abc) -> Switch4/3
  EnClosedLoop/1 -> Closed Loop Control/Enable, Switch4/2, NOT/1

== system pulse_heating_official_spine_v04_git_recovery/PMSMDriveThermal_Inverter_And_Motor/Encoder ==
  Ideal Rotational Motion Sensor : fl_lib/Mechanical/Mechanical Sensors/Ideal Rotational Motion Sensor  reference=foundation.enum.MeasurementReference.difference  acceleration_port=false  velocity_port=true  position_port=true  wrap_angle=simscape.enum.onoff.off  offset=0 deg
  Ideal Torque Sensor : fl_lib/Mechanical/Mechanical Sensors/Ideal Torque Sensor
  Mux : Mux  Inputs=2
  PS-Simulink Converter : nesl_utility/PS-Simulink Converter  PhysicalDomain=network_engine_domain  SubClassName=ps_output  LeftPortType=input  RightPortType=output  PseudoPeriodic=off  Frequencies=[]  VectorFormat=1-D array  Unit=rad/s  AffineConversion=off
  PS-Simulink Converter1 : nesl_utility/PS-Simulink Converter  PhysicalDomain=network_engine_domain  SubClassName=ps_output  LeftPortType=input  RightPortType=output  PseudoPeriodic=off  Frequencies=[]  VectorFormat=1-D array  Unit=rad  AffineConversion=off
  PS-Simulink Converter2 : nesl_utility/PS-Simulink Converter  PhysicalDomain=network_engine_domain  SubClassName=ps_output  LeftPortType=input  RightPortType=output  PseudoPeriodic=off  Frequencies=[]  VectorFormat=1-D array  Unit=N*m  AffineConversion=off
  1L : PMIOPort  Side=Left
  2L : PMIOPort  Port=2  Side=Left
  1R : PMIOPort  Port=3  Side=Right
  2R : PMIOPort  Port=4  Side=Right
  meas : Outport  VectorParamsAs1DForOutWhenUnconnected=off
  tag scope: trqMotor=global, wMotor=global
  wires:
  PS-Simulink Converter/1 -> Mux/1, [wMotor]
  PS-Simulink Converter1/1 -> Mux/2
  Mux/1 -> meas/1
  PS-Simulink Converter2/1 -> [trqMotor]
  connections:
  Ideal Rotational Motion Sensor/RConn3 -- PS-Simulink Converter1/LConn1
  Ideal Rotational Motion Sensor/RConn2 -- PS-Simulink Converter/LConn1
  Ideal Torque Sensor/RConn1 -- 1R/RConn1 -- Ideal Rotational Motion Sensor/LConn1
  Ideal Rotational Motion Sensor/RConn1 -- 2L/RConn1 -- 2R/RConn1
  1L/RConn1 -- Ideal Torque Sensor/LConn1
  Ideal Torque Sensor/RConn2 -- PS-Simulink Converter2/LConn1

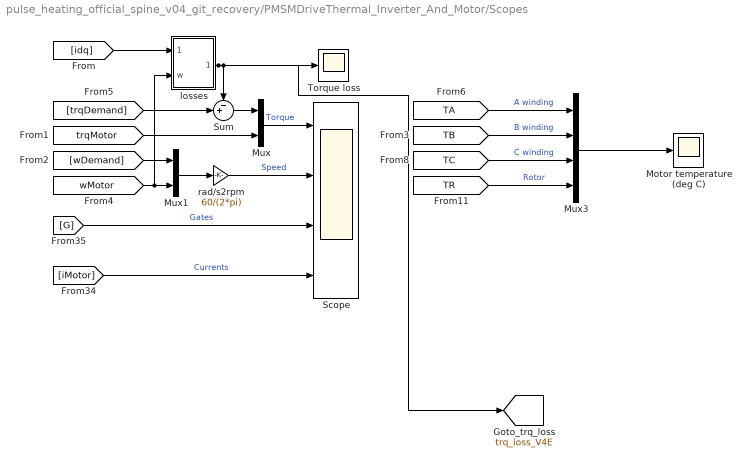
== system pulse_heating_official_spine_v04_git_recovery/PMSMDriveThermal_Inverter_And_Motor/Scopes ==
  Motor temperature (deg C) : Scope
      settings: Title=Motor temperature (deg C)  ActiveDisplayYMinimum=24.92686  ActiveDisplayYMaximum=25.65828  DataLoggingMaxPoints=500000  DataLoggingDecimation=10
  Mux : Mux  Inputs=2
  Mux1 : Mux  Inputs=2
  Mux3 : Mux
  Scope : Scope  NumInputPorts=4
      settings: Title=Demanded and achieved torques  ActiveDisplayYMinimum=-8.43651  ActiveDisplayYMaximum=36.34769
  Sum : Sum  Inputs=-+|
  Torque loss : Scope
      settings: ActiveDisplayYMinimum=-0.64352  ActiveDisplayYMaximum=5.79171
  losses : Subsystem
  rad/s2rpm : Gain  Gain=60/(2*pi)
  tag scope: trq_loss_V4E=global
  wires:
  [trqDemand] -> Sum/2
  Sum/1 -> Mux/1
  losses/1(tq_loss) -> Sum/1, Torque loss/1, [trq_loss_V4E]
  [idq] -> losses/1(idq)
  Mux/1 -> Scope/1  "Torque"
  Mux1/1 -> rad/s2rpm/1
  [trqMotor] -> Mux/2
  [iMotor] -> Scope/4  "Currents"
  [wMotor] -> Mux1/2, losses/2(w)
  [wDemand] -> Mux1/1
  [G] -> Scope/3  "Gates"
  rad/s2rpm/1 -> Scope/2  "Speed"
  Mux3/1 -> Motor temperature (deg C)/1
  [TA] -> Mux3/1  "A winding"
  [TB] -> Mux3/2  "B winding"
  [TR] -> Mux3/4  "Rotor"
  [TC] -> Mux3/3  "C winding"

== system pulse_heating_official_spine_v04_git_recovery/PMSMDriveThermal_Inverter_And_Motor/Sensing currents ==
  Current Sensor : ee_lib/Sensors & Transducers/Current Sensor (Three-Phase)
  PS-Simulink Converter : nesl_utility/PS-Simulink Converter  PhysicalDomain=network_engine_domain  SubClassName=ps_output  LeftPortType=input  RightPortType=output  PseudoPeriodic=off  Frequencies=[]  VectorFormat=1-D array  Unit=A  AffineConversion=off
  Conn1 : PMIOPort  Side=Left
  Conn2 : PMIOPort  Port=2  Side=Right
  tag scope: i=global
  wires:
  PS-Simulink Converter/1 -> [i]
  connections:
  Current Sensor/LConn1 -- Conn1/RConn1
  Conn2/RConn1 -- Current Sensor/RConn2
  Current Sensor/RConn1 -- PS-Simulink Converter/LConn1

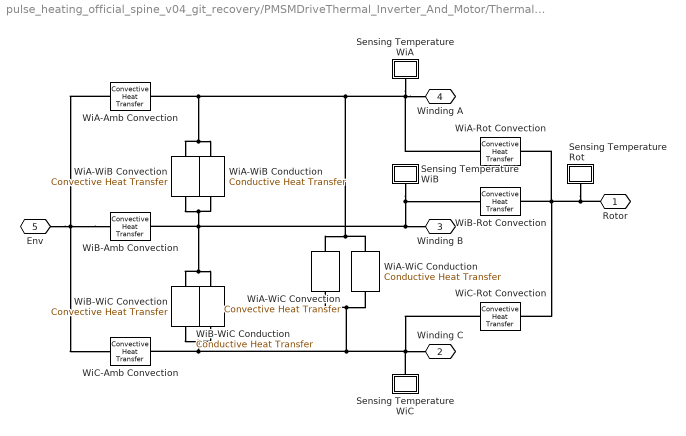
== system pulse_heating_official_spine_v04_git_recovery/PMSMDriveThermal_Inverter_And_Motor/Thermal model ==
  Sensing Temperature Rot : Subsystem
      mask Display: disp('TR')
  Sensing Temperature WiA : Subsystem
      mask Display: disp('TA')
  Sensing Temperature WiB : Subsystem
      mask Display: disp('TB')
  Sensing Temperature WiC : Subsystem
      mask Display: disp('TC')
  WiA-Amb Convection : fl_lib/Thermal/Thermal Elements/Convective Heat Transfer  thermal_type=foundation.enum.constant_variable.constant  area=0.1 m^2  heat_tr_coeff=20 W/(m^2 * K)  min_heat_tr_coeff=1e-3 W/(K*m^2)  T_specify=off  T_priority=None  T=0 K  T_nominal_specify=off  T_nominal_value=1  T_nominal_unit=K  Q_specify=off  Q_priority=None  Q=0 J/s  Q_nominal_specify=off  Q_nominal_value=1  Q_nominal_unit=J/s
  WiA-Rot Convection : fl_lib/Thermal/Thermal Elements/Convective Heat Transfer  thermal_type=foundation.enum.constant_variable.constant  area=0.02 m^2  heat_tr_coeff=200 W/(m^2 * K)  min_heat_tr_coeff=1e-3 W/(K*m^2)  T_specify=off  T_priority=None  T=0 K  T_nominal_specify=off  T_nominal_value=1  T_nominal_unit=K  Q_specify=off  Q_priority=None  Q=0 J/s  Q_nominal_specify=off  Q_nominal_value=1  Q_nominal_unit=J/s
  WiA-WiB Conduction : fl_lib/Thermal/Thermal Elements/Conductive Heat Transfer  thermal_type=foundation.enum.ConstantVariableTabulated.Constant  wall_geometry=foundation.enum.ConductionWallGeometry.Planar  area=0.002 m^2  thickness=0.1 m  d_in=0.05 m  d_out=0.1 m  L=1 m  th_cond_min=10 W/(K*m)  th_cond=80 W/(m*K)  th_cond_TLU=[413, 401, 392, 383, 371, 357, 342] W/(K*m)  temp_TLU=[200, 273, 400, 600, 800, 1000, 1200] K  T_specify=off  T_priority=None  T=0 K  T_nominal_specify=off  T_nominal_value=1  T_nominal_unit=K  Q_specify=off  Q_priority=None  Q=0 J/s  Q_nominal_specify=off  Q_nominal_value=1  Q_nominal_unit=J/s
  WiA-WiB Convection : fl_lib/Thermal/Thermal Elements/Convective Heat Transfer  thermal_type=foundation.enum.constant_variable.constant  area=0.004 m^2  heat_tr_coeff=200 W/(m^2 * K)  min_heat_tr_coeff=1e-3 W/(K*m^2)  T_specify=off  T_priority=None  T=0 K  T_nominal_specify=off  T_nominal_value=1  T_nominal_unit=K  Q_specify=off  Q_priority=None  Q=0 J/s  Q_nominal_specify=off  Q_nominal_value=1  Q_nominal_unit=J/s
  WiA-WiC Conduction : fl_lib/Thermal/Thermal Elements/Conductive Heat Transfer  thermal_type=foundation.enum.ConstantVariableTabulated.Constant  wall_geometry=foundation.enum.ConductionWallGeometry.Planar  area=0.002 m^2  thickness=0.1 m  d_in=0.05 m  d_out=0.1 m  L=1 m  th_cond_min=10 W/(K*m)  th_cond=80 W/(m*K)  th_cond_TLU=[413, 401, 392, 383, 371, 357, 342] W/(K*m)  temp_TLU=[200, 273, 400, 600, 800, 1000, 1200] K  T_specify=off  T_priority=None  T=0 K  T_nominal_specify=off  T_nominal_value=1  T_nominal_unit=K  Q_specify=off  Q_priority=None  Q=0 J/s  Q_nominal_specify=off  Q_nominal_value=1  Q_nominal_unit=J/s
  WiA-WiC Convection : fl_lib/Thermal/Thermal Elements/Convective Heat Transfer  thermal_type=foundation.enum.constant_variable.constant  area=0.004 m^2  heat_tr_coeff=200 W/(m^2 * K)  min_heat_tr_coeff=1e-3 W/(K*m^2)  T_specify=off  T_priority=None  T=0 K  T_nominal_specify=off  T_nominal_value=1  T_nominal_unit=K  Q_specify=off  Q_priority=None  Q=0 J/s  Q_nominal_specify=off  Q_nominal_value=1  Q_nominal_unit=J/s
  WiB-Amb Convection : fl_lib/Thermal/Thermal Elements/Convective Heat Transfer  thermal_type=foundation.enum.constant_variable.constant  area=0.1 m^2  heat_tr_coeff=20 W/(m^2 * K)  min_heat_tr_coeff=1e-3 W/(K*m^2)  T_specify=off  T_priority=None  T=0 K  T_nominal_specify=off  T_nominal_value=1  T_nominal_unit=K  Q_specify=off  Q_priority=None  Q=0 J/s  Q_nominal_specify=off  Q_nominal_value=1  Q_nominal_unit=J/s
  WiB-Rot Convection : fl_lib/Thermal/Thermal Elements/Convective Heat Transfer  thermal_type=foundation.enum.constant_variable.constant  area=0.02 m^2  heat_tr_coeff=200 W/(m^2 * K)  min_heat_tr_coeff=1e-3 W/(K*m^2)  T_specify=off  T_priority=None  T=0 K  T_nominal_specify=off  T_nominal_value=1  T_nominal_unit=K  Q_specify=off  Q_priority=None  Q=0 J/s  Q_nominal_specify=off  Q_nominal_value=1  Q_nominal_unit=J/s
  WiB-WiC Conduction : fl_lib/Thermal/Thermal Elements/Conductive Heat Transfer  thermal_type=foundation.enum.ConstantVariableTabulated.Constant  wall_geometry=foundation.enum.ConductionWallGeometry.Planar  area=0.002 m^2  thickness=0.1 m  d_in=0.05 m  d_out=0.1 m  L=1 m  th_cond_min=10 W/(K*m)  th_cond=80 W/(m*K)  th_cond_TLU=[413, 401, 392, 383, 371, 357, 342] W/(K*m)  temp_TLU=[200, 273, 400, 600, 800, 1000, 1200] K  T_specify=off  T_priority=None  T=0 K  T_nominal_specify=off  T_nominal_value=1  T_nominal_unit=K  Q_specify=off  Q_priority=None  Q=0 J/s  Q_nominal_specify=off  Q_nominal_value=1  Q_nominal_unit=J/s
  WiB-WiC Convection : fl_lib/Thermal/Thermal Elements/Convective Heat Transfer  thermal_type=foundation.enum.constant_variable.constant  area=0.004 m^2  heat_tr_coeff=200 W/(m^2 * K)  min_heat_tr_coeff=1e-3 W/(K*m^2)  T_specify=off  T_priority=None  T=0 K  T_nominal_specify=off  T_nominal_value=1  T_nominal_unit=K  Q_specify=off  Q_priority=None  Q=0 J/s  Q_nominal_specify=off  Q_nominal_value=1  Q_nominal_unit=J/s
  WiC-Amb Convection : fl_lib/Thermal/Thermal Elements/Convective Heat Transfer  thermal_type=foundation.enum.constant_variable.constant  area=0.1 m^2  heat_tr_coeff=20 W/(m^2 * K)  min_heat_tr_coeff=1e-3 W/(K*m^2)  T_specify=off  T_priority=None  T=0 K  T_nominal_specify=off  T_nominal_value=1  T_nominal_unit=K  Q_specify=off  Q_priority=None  Q=0 J/s  Q_nominal_specify=off  Q_nominal_value=1  Q_nominal_unit=J/s
  WiC-Rot Convection : fl_lib/Thermal/Thermal Elements/Convective Heat Transfer  thermal_type=foundation.enum.constant_variable.constant  area=0.02 m^2  heat_tr_coeff=200 W/(m^2 * K)  min_heat_tr_coeff=1e-3 W/(K*m^2)  T_specify=off  T_priority=None  T=0 K  T_nominal_specify=off  T_nominal_value=1  T_nominal_unit=K  Q_specify=off  Q_priority=None  Q=0 J/s  Q_nominal_specify=off  Q_nominal_value=1  Q_nominal_unit=J/s
  Rotor : PMIOPort  Side=Left
  Winding C : PMIOPort  Port=2  Side=Right
  Winding B : PMIOPort  Port=3  Side=Right
  Winding A : PMIOPort  Port=4  Side=Right
  Env : PMIOPort  Port=5  Side=Left
  connections:
  WiB-Amb Convection/RConn1 -- WiC-Amb Convection/RConn1 -- Env/RConn1 -- WiA-Amb Convection/RConn1
  Sensing Temperature WiC/LConn1 -- WiA-WiC Conduction/LConn1 -- WiA-WiC Convection/LConn1 -- WiC-Amb Convection/LConn1 -- WiB-WiC Convection/RConn1 -- WiB-WiC Conduction/RConn1 -- Winding C/RConn1 -- WiC-Rot Convection/RConn1
  WiB-WiC Convection/LConn1 -- WiB-WiC Conduction/LConn1 -- WiB-Amb Convection/LConn1 -- Winding B/RConn1 -- WiB-Rot Convection/RConn1 -- Sensing Temperature WiB/LConn1 -- WiA-WiB Conduction/RConn1 -- WiA-WiB Convection/RConn1
  WiA-Rot Convection/LConn1 -- WiB-Rot Convection/LConn1 -- WiC-Rot Convection/LConn1 -- Sensing Temperature Rot/LConn1 -- Rotor/RConn1
  Winding A/RConn1 -- Sensing Temperature WiA/LConn1 -- WiA-Amb Convection/LConn1 -- WiA-WiB Conduction/LConn1 -- WiA-WiB Convection/LConn1 -- WiA-WiC Convection/RConn1 -- WiA-WiC Conduction/RConn1 -- WiA-Rot Convection/RConn1
